simulink model "Pacemaker_A2"  (R2022b)
settings: Solver=FixedStepAuto  StartTime=0.0  StopTime=10.0  FixedStep=1e-3  RelTol=1e-3  EnableMultiTasking=on
undefined symbols (not defined in the file): A0, A1, D0, D1, D10, D11, D12, D13, D2, D3, D5, D6, D8, D9, magnitude, PTA0, PTA1, PTA2, PTB2, PTB3, PTB9, PTC16, PTC17, PTC2, PTC4, PTD0, PTD1, PTD2, PTD3
libraries: frdmk64flib x19, etargetslib x18, dspstat3 x1
settings Model: SimulationMode=external  ExtModeTrigDuration=5  Creator=27161  LastModifiedBy=27161
settings SolverCC: AlgebraicLoopSolver=TrustRegion
settings OptimizationCC: EnhancedBackFolding=on  PassReuseOutputArgsAs=Individual arguments  ZeroExternalMemoryAtStartup=off  ZeroInternalMemoryAtStartup=off  MaxStackSize=64  OptimizeBlockOrder=speed  DifferentSizesBufferReuse=on  OptimizationCustomize=off  EfficientTunableParamExpr=on
settings DebuggingCC: ParameterTunabilityLossMsg=error  UnconnectedInputMsg=warning  UnconnectedOutputMsg=warning  UnconnectedLineMsg=warning  SFMachineParentedDataDiag=warning
settings HardwareCC: ProdBitPerPointer=32  ProdBitPerSizeT=32  ProdBitPerPtrDiffT=32  ProdLargestAtomicInteger=Long  ProdLargestAtomicFloat=Double  ProdWordSize=32  ProdHWDeviceType=ARM Compatible->ARM Cortex
settings ModelReferenceCC: EnableRefExpFcnMdlSchedulingChecks=on
settings SFSimCC: MATLABDynamicMemAlloc=off
settings RTWCC: Description=Embedded Coder  SystemTargetFile=ert.tlc  HardwareBoard=NXP FRDM-K64F  TLCOptions="-aInlineSetEventsForThisBaseRateFcn=TLC_FALSE -aSuppressMultiTaskScheduler=TLC_FALSE  -aRateBasedStepFcn=0"  TemplateMakefile=ert_default_tmf  Toolchain=GNU Tools for ARM Embedded Processors
settings CodeAppCC: ForceParamTrailComments=on  IgnoreCustomStorageClasses=off  OperatorAnnotations=on  SimulinkDataObjDesc=on  SFDataObjDesc=on  InsertBlockDesc=on
settings ERTTargetCC: ExtMode=on  ExtModeTransport=4  ExtModeMexFile=sendToCommService  ExtModeMexArgs='Pacemaker_A2' 0

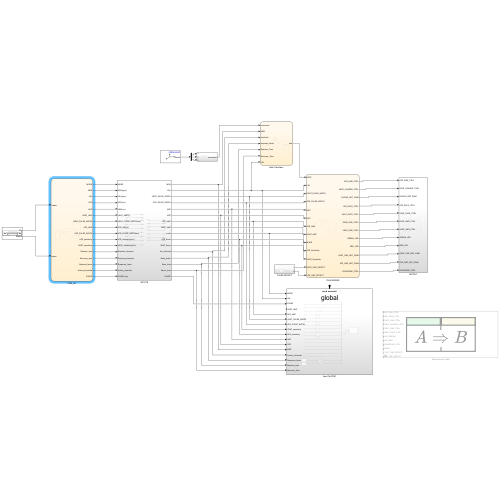
[thumbnail: Simulink's stored preview of the top-level diagram]
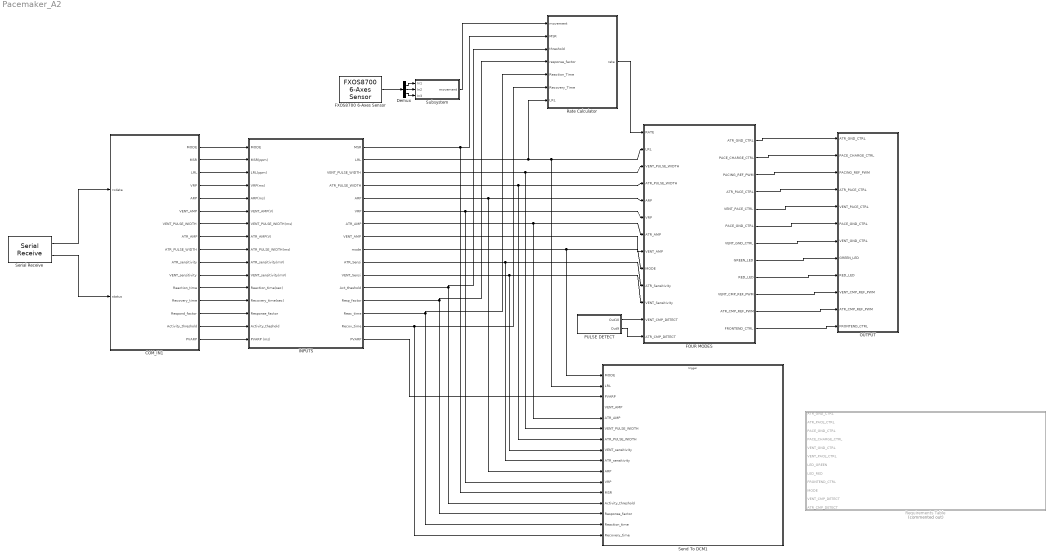
== system Pacemaker_A2 ==
  COM_IN1 : Stateflow chart  TreatAsAtomicUnit=on
      settings: PortSchema="{\"entries\":[{\"content\":{\"sides\":[{\"content\":{\"connectorIds\":[\"In1\",\"In2\"]},\"type\":\"ConnectorPlacement.EquallySpacedRectSide\",\"uuid\":\"bacdf752-87eb-4404-babc-2d3eecd8d2c0\"},{\"content\":{\"connectorIds\":[\"Out12\",\"Out8\",\"Out1\",\"Out2\",\"Out3\",\"Out4\",\"Out5\",\"Out6\",\"Out7\",\"Out9\",\"Out10\",\"Out13\",\"Out14\",\"Out15\",\"Out16\",\"Out11\"],\"side\":\"RIGHT\"},\"type\":\"ConnectorPlacement.EquallySpacedRectSide\",\"uuid\":\"87a5995d-41f9-45bd-b026-59ec7d01c35a\"},{\"content\":{\"connectorIds\":[],\"side\":\"TOP\"},\"type\":\"ConnectorPlacement.EquallySpacedRectSide\",\"uuid\":\"9c1d1ff9-71c1-4ac7-ac77-ae13538ca481\"}]},\"type\":\"ConnectorPlacement.EquallySpacedConnector\",\"uuid\":\"f58684e7-fbf2-4992-a059-d31a56d65e02\"}],\"packageUris\":[\"http://schema.mathworks.com/mf0/Connector/R2020b\"],\"version\":\"1.0\"}"
  Demux : Demux  Outputs=3
  FOUR MODES : Stateflow chart  TreatAsAtomicUnit=on
      settings: PortSchema="{\"entries\":[{\"content\":{\"sides\":[{\"content\":{\"connectorIds\":[\"In11\",\"In8\",\"In2\",\"In1\",\"In9\",\"In10\",\"In5\",\"In4\",\"In6\",\"In13\",\"In12\",\"In3\",\"In7\"]},\"type\":\"ConnectorPlacement.EquallySpacedRectSide\",\"uuid\":\"6661be6b-aedb-4592-878a-fd9116f5820d\"},{\"content\":{\"connectorIds\":[\"Out7\",\"Out1\",\"Out2\",\"Out3\",\"Out4\",\"Out6\",\"Out5\",\"Out9\",\"Out10\",\"Out11\",\"Out12\",\"Out8\"],\"side\":\"RIGHT\"},\"type\":\"ConnectorPlacement.EquallySpacedRectSide\",\"uuid\":\"f16586c3-0c99-4971-ba5f-75b93d25059c\"},{\"content\":{\"connectorIds\":[],\"side\":\"TOP\"},\"type\":\"ConnectorPlacement.EquallySpacedRectSide\",\"uuid\":\"27cb1bd0-c170-4ecc-a4df-3797e7aecef3\"}]},\"type\":\"ConnectorPlacement.EquallySpacedConnector\",\"uuid\":\"03557791-41f4-4916-8cde-1fcab0cf663d\"}],\"packageUris\":[\"http://schema.mathworks.com/mf0/Connector/R2020b\"],\"version\":\"1.0\"}"
  FXOS8700 6-Axes Sensor : frdmk64flib/FXOS8700 6-Axes Sensor  Activesensor=Accelerometer only  ODR=800Hz  HybridODR=400Hz  Accelfullrange=-4g to +4g  SampleTime=-1
  INPUTS : Subsystem
  OUTPUT : Subsystem
  PULSE DETECT : Subsystem
  Rate Calculator : Stateflow chart  TreatAsAtomicUnit=on
      settings: PortSchema="{\"entries\":[{\"content\":{\"sides\":[{\"content\":{\"connectorIds\":[\"In3\",\"In7\",\"In5\",\"In4\",\"In1\",\"In2\",\"In6\"]},\"type\":\"ConnectorPlacement.EquallySpacedRectSide\",\"uuid\":\"c5d5357b-99af-427e-a4c2-6249b97164da\"},{\"content\":{\"connectorIds\":[\"Out1\"],\"side\":\"RIGHT\"},\"type\":\"ConnectorPlacement.EquallySpacedRectSide\",\"uuid\":\"358f3739-9c7f-4556-a3f3-e36ee066d1ea\"},{\"content\":{\"connectorIds\":[],\"side\":\"TOP\"},\"type\":\"ConnectorPlacement.EquallySpacedRectSide\",\"uuid\":\"e7873f65-b91d-40fa-bd89-8dce436ca138\"}]},\"type\":\"ConnectorPlacement.EquallySpacedConnector\",\"uuid\":\"f1b9a7e0-0d96-4ba5-9c87-c58b64bb2144\"}],\"packageUris\":[\"http://schema.mathworks.com/mf0/Connector/R2020b\"],\"version\":\"1.0\"}"
  Requirements Table : Requirements Table  Commented=on  TreatAsAtomicUnit=on
  Send To DCM1 : Subsystem
  Serial Receive : frdmk64flib/Serial Receive  SCIModule=0  Baudrate=uint32(9600)  Parity=None  StopBits=1  HardwareFlowControl=None  ByteOrder=LittleEndian  DataType=uint8  DataLength=10  BlockingMode=off  OutputStatus=on  SampleTime=0.1
  Subsystem : Subsystem
  wires:
  FOUR MODES/7(ATR_GND_CTRL) -> OUTPUT/1(ATR_GND_CTRL)
  FOUR MODES/1(PACE_CHARGE_CTRL) -> OUTPUT/2(PACE_CHARGE_CTRL)
  FOUR MODES/2(PACING_REF_PWM) -> OUTPUT/3(PACING_REF_PWM)
  FOUR MODES/3(ATR_PACE_CTRL) -> OUTPUT/4(ATR_PACE_CTRL)
  FOUR MODES/4(VENT_PACE_CTRL) -> OUTPUT/5(VENT_PACE_CTRL)
  FOUR MODES/5(VENT_GND_CTRL) -> OUTPUT/7(VENT_GND_CTRL)
  FOUR MODES/6(PACE_GND_CTRL) -> OUTPUT/6(PACE_GND_CTRL)
  FOUR MODES/9(GREEN_LED) -> OUTPUT/8(GREEN_LED)
  FOUR MODES/12(ATR_CMP_REF_PWM) -> OUTPUT/11(ATR_CMP_REF_PWM)
  FOUR MODES/11(VENT_CMP_REF_PWM) -> OUTPUT/10(VENT_CMP_REF_PWM)
  FOUR MODES/10(RED_LED) -> OUTPUT/9(RED_LED)
  FOUR MODES/8(FRONTEND_CTRL) -> OUTPUT/12(FRONTEND_CTRL)
  PULSE DETECT/2(Out9) -> FOUR MODES/7(ATR_CMP_DETECT)
  PULSE DETECT/1(Out10) -> FOUR MODES/3(VENT_CMP_DETECT)
  Demux/3 -> Subsystem/3(In3)
  Subsystem/1(movement) -> Rate Calculator/3(movement)
  Demux/1 -> Subsystem/1(In1)
  FXOS8700 6-Axes Sensor/1 -> Demux/1
  Demux/2 -> Subsystem/2(In2)
  COM_IN1/12(MODE) -> INPUTS/1(MODE)
  COM_IN1/1(LRL) -> INPUTS/3(LRL(ppm))
  COM_IN1/2(VRP) -> INPUTS/4(VRP(ms))
  COM_IN1/3(ARP) -> INPUTS/5(ARP(ms))
  COM_IN1/4(VENT_AMP) -> INPUTS/6(VENT_AMP(V))
  COM_IN1/5(VENT_PULSE_WIDTH) -> INPUTS/7(VENT_PULSE_WIDTH(ms))
  COM_IN1/6(ATR_AMP) -> INPUTS/8(ATR_AMP(V))
  COM_IN1/7(ATR_PULSE_WIDTH) -> INPUTS/9(ATR_PULSE_WIDTH(ms))
  COM_IN1/8(MSR) -> INPUTS/2(MSR(ppm))
  COM_IN1/9(ATR_sensitivity) -> INPUTS/10(ATR_sensitivity(mV))
  COM_IN1/10(VENT_sensitivity) -> INPUTS/11(VENT_sensitivity(mV))
  COM_IN1/13(Reaction_time) -> INPUTS/12(Reaction_time(sec))
  COM_IN1/14(Recovery_time) -> INPUTS/13(Recovery_time(sec))
  COM_IN1/11(PVARP) -> INPUTS/16(PVARP (ms))
  Serial Receive/1 -> COM_IN1/1(rxdata)
  Serial Receive/2 -> COM_IN1/2(status)
  COM_IN1/15(Respond_factor) -> INPUTS/14(Response_factor)
  COM_IN1/16(Activity_threshold) -> INPUTS/15(Activity_theshold)
  INPUTS/2(LRL) -> FOUR MODES/8(LRL), Send To DCM1/2(LRL), Rate Calculator/6(LRL)
  INPUTS/1(MSR) -> Rate Calculator/7(MSR), Send To DCM1/12(MSR)
  INPUTS/3(VENT_PULSE_WIDTH) -> FOUR MODES/2(VENT_PULSE_WIDTH), Send To DCM1/6(VENT_PULSE_WIDTH)
  INPUTS/4(ATR_PULSE_WIDTH) -> FOUR MODES/1(ATR_PULSE_WIDTH), Send To DCM1/7(ATR_PULSE_WIDTH)
  INPUTS/5(ARP) -> Send To DCM1/10(ARP), FOUR MODES/9(ARP)
  INPUTS/6(VRP) -> Send To DCM1/11(VRP), FOUR MODES/10(VRP)
  INPUTS/7(ATR_AMP) -> Send To DCM1/5(ATR_AMP), FOUR MODES/5(ATR_AMP)
  INPUTS/8(VENT_AMP) -> FOUR MODES/4(VENT_AMP)
  INPUTS/9(mode) -> Send To DCM1/1(MODE), FOUR MODES/6(MODE)
  INPUTS/14(Reac_time) -> Rate Calculator/1(Reaction_Time), Send To DCM1/15(Reaction_time)
  INPUTS/15(Recov_time) -> Rate Calculator/2(Recovery_Time), Send To DCM1/16(Recovery_time)
  INPUTS/12(Act_theshold) -> Rate Calculator/5(threshold), Send To DCM1/13(Activity_threshold)
  INPUTS/13(Resp_factor) -> Rate Calculator/4(response_factor), Send To DCM1/14(Response_factor)
  INPUTS/10(ATR_Sensi) -> Send To DCM1/9(ATR_sensitivity), FOUR MODES/13(ATR_Sensitivity)
  INPUTS/11(VENT_Sensi) -> Send To DCM1/8(VENT_sensitivity), FOUR MODES/12(VENT_Sensitivity)
  Rate Calculator/1(rate) -> FOUR MODES/11(RATE)
  INPUTS/16(PVARP) -> Send To DCM1/3(PVARP)

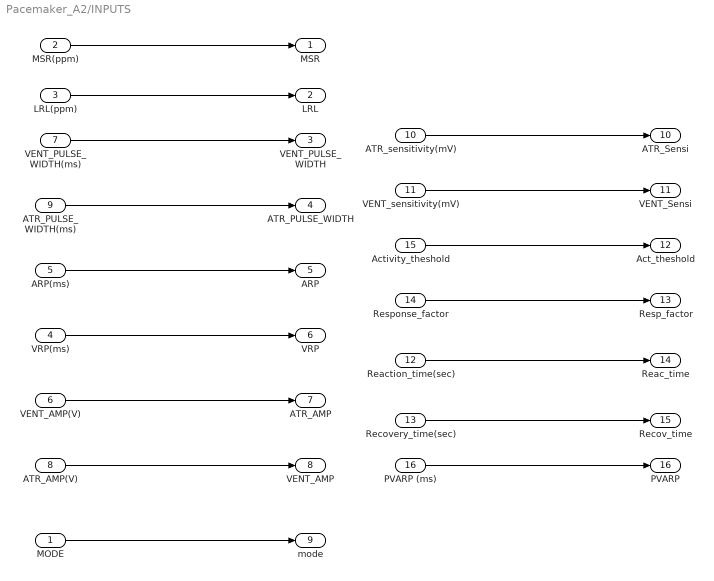
== system Pacemaker_A2/INPUTS ==
  MODE : Inport
  MSR(ppm) : Inport  Port=2
  LRL(ppm) : Inport  Port=3
  VRP(ms) : Inport  Port=4
  ARP(ms) : Inport  Port=5
  VENT_AMP(V) : Inport  Port=6
  VENT_PULSE_WIDTH(ms) : Inport  Port=7
  ATR_AMP(V) : Inport  Port=8
  ATR_PULSE_WIDTH(ms) : Inport  Port=9
  ATR_sensitivity(mV) : Inport  Port=10
  VENT_sensitivity(mV) : Inport  Port=11
  Reaction_time(sec) : Inport  Port=12
  Recovery_time(sec) : Inport  Port=13
  Response_factor : Inport  Port=14
  Activity_theshold : Inport  Port=15
  PVARP (ms) : Inport  Port=16
  MSR : Outport
  LRL : Outport  Port=2
  VENT_PULSE_WIDTH : Outport  Port=3
  ATR_PULSE_WIDTH : Outport  Port=4
  ARP : Outport  Port=5
  VRP : Outport  Port=6
  ATR_AMP : Outport  Port=7
  VENT_AMP : Outport  Port=8
  mode : Outport  Port=9
  ATR_Sensi : Outport  Port=10
  VENT_Sensi : Outport  Port=11
  Act_theshold : Outport  Port=12
  Resp_factor : Outport  Port=13
  Reac_time : Outport  Port=14
  Recov_time : Outport  Port=15
  PVARP : Outport  Port=16
  wires:
  LRL(ppm)/1 -> LRL/1
  VENT_PULSE_WIDTH(ms)/1 -> VENT_PULSE_WIDTH/1
  ATR_PULSE_WIDTH(ms)/1 -> ATR_PULSE_WIDTH/1
  ARP(ms)/1 -> ARP/1
  VRP(ms)/1 -> VRP/1
  VENT_AMP(V)/1 -> ATR_AMP/1
  ATR_AMP(V)/1 -> VENT_AMP/1
  MODE/1 -> mode/1
  MSR(ppm)/1 -> MSR/1
  ATR_sensitivity(mV)/1 -> ATR_Sensi/1
  VENT_sensitivity(mV)/1 -> VENT_Sensi/1
  Activity_theshold/1 -> Act_theshold/1
  Response_factor/1 -> Resp_factor/1
  Reaction_time(sec)/1 -> Reac_time/1
  Recovery_time(sec)/1 -> Recov_time/1
  PVARP (ms)/1 -> PVARP/1

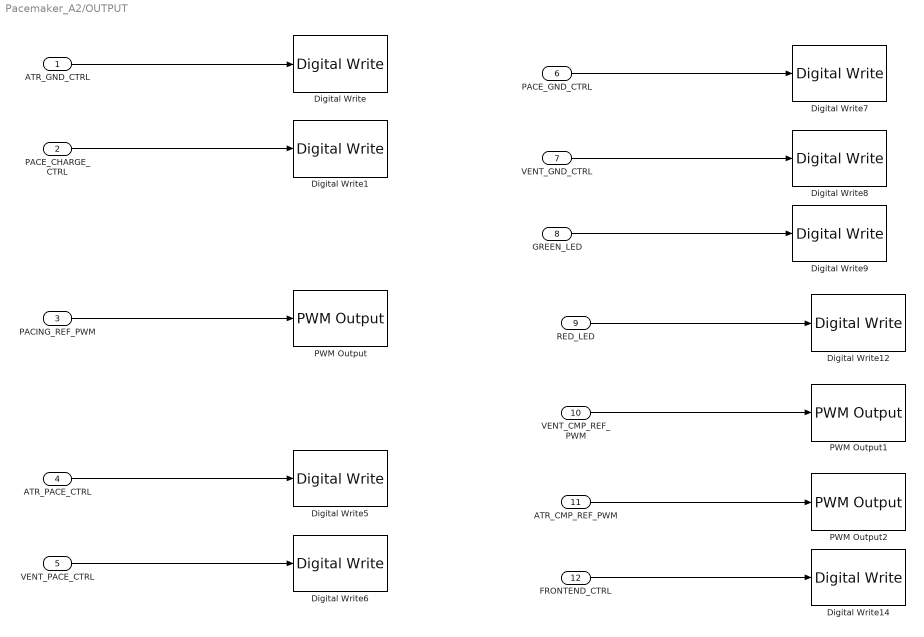
== system Pacemaker_A2/OUTPUT ==
  ATR_GND_CTRL : Inport
  PACE_CHARGE_CTRL : Inport  Port=2
  PACING_REF_PWM : Inport  Port=3
  ATR_PACE_CTRL : Inport  Port=4
  VENT_PACE_CTRL : Inport  Port=5
  PACE_GND_CTRL : Inport  Port=6
  VENT_GND_CTRL : Inport  Port=7
  GREEN_LED : Inport  Port=8
  RED_LED : Inport  Port=9
  VENT_CMP_REF_PWM : Inport  Port=10
  ATR_CMP_REF_PWM : Inport  Port=11
  FRONTEND_CTRL : Inport  Port=12
  Digital Write : frdmk64flib/Digital Write  Whichpin=PTD2 (D11)
  Digital Write1 : frdmk64flib/Digital Write  Whichpin=PTB9 (D2)
  Digital Write12 : frdmk64flib/Digital Write  Whichpin=RED_LED
  Digital Write14 : frdmk64flib/Digital Write  Whichpin=PTD1 (D13)
  Digital Write5 : frdmk64flib/Digital Write  Whichpin=PTA0 (D8)
  Digital Write6 : frdmk64flib/Digital Write  Whichpin=PTC4 (D9)
  Digital Write7 : frdmk64flib/Digital Write  Whichpin=PTD0 (D10)
  Digital Write8 : frdmk64flib/Digital Write  Whichpin=PTD3 (D12)
  Digital Write9 : frdmk64flib/Digital Write  Whichpin=GREEN_LED
  PWM Output : frdmk64flib/PWM Output  Whichpin=PTA2 (D5)  InitialFrequency=2000  InitialDutyCycle=0
  PWM Output1 : frdmk64flib/PWM Output  Whichpin=PTA1 (D3)  InitialFrequency=2000  InitialDutyCycle=0
  PWM Output2 : frdmk64flib/PWM Output  Whichpin=PTC2 (D6)  InitialFrequency=2000  InitialDutyCycle=0
  wires:
  ATR_GND_CTRL/1 -> Digital Write/1
  PACE_CHARGE_CTRL/1 -> Digital Write1/1
  PACING_REF_PWM/1 -> PWM Output/1
  ATR_PACE_CTRL/1 -> Digital Write5/1
  VENT_PACE_CTRL/1 -> Digital Write6/1
  PACE_GND_CTRL/1 -> Digital Write7/1
  VENT_GND_CTRL/1 -> Digital Write8/1
  GREEN_LED/1 -> Digital Write9/1
  ATR_CMP_REF_PWM/1 -> PWM Output2/1
  VENT_CMP_REF_PWM/1 -> PWM Output1/1
  RED_LED/1 -> Digital Write12/1
  FRONTEND_CTRL/1 -> Digital Write14/1

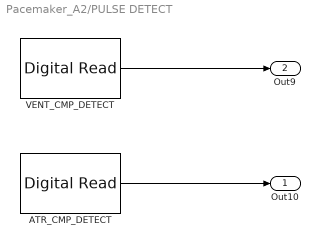
== system Pacemaker_A2/PULSE DETECT ==
  ATR_CMP_DETECT : frdmk64flib/Digital Read  Whichpin=PTC16 (D0)  SampleTime=-1
  VENT_CMP_DETECT : frdmk64flib/Digital Read  Whichpin=PTC17 (D1)  SampleTime=-1
  Out10 : Outport
  Out9 : Outport  Port=2
  wires:
  VENT_CMP_DETECT/1 -> Out9/1
  ATR_CMP_DETECT/1 -> Out10/1

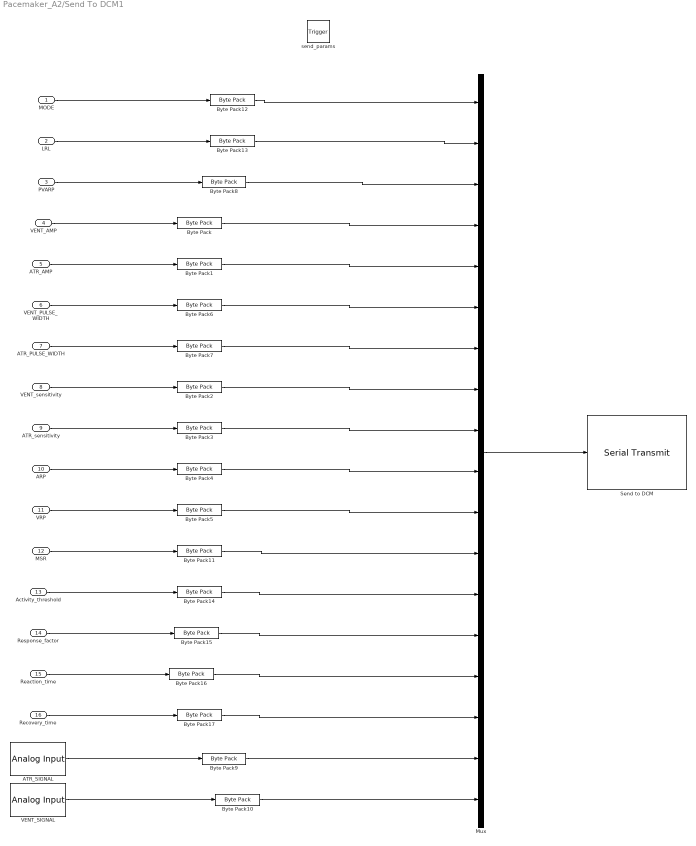
== system Pacemaker_A2/Send To DCM1 ==
  MODE : Inport
  LRL : Inport  Port=2
  PVARP : Inport  Port=3
  VENT_AMP : Inport  Port=4
  ATR_AMP : Inport  Port=5
  VENT_PULSE_WIDTH : Inport  Port=6
  ATR_PULSE_WIDTH : Inport  Port=7
  VENT_sensitivity : Inport  Port=8
  ATR_sensitivity : Inport  Port=9
  ARP : Inport  Port=10
  VRP : Inport  Port=11
  MSR : Inport  Port=12
  Activity_threshold : Inport  Port=13
  Response_factor : Inport  Port=14
  Reaction_time : Inport  Port=15
  Recovery_time : Inport  Port=16
  send_params : TriggerPort  TriggerType=function-call  IsSimulinkFunction=on  FunctionName=send_params  VariantControl=(inherit)  PortDimensions=1
  ATR_SIGNAL : frdmk64flib/Analog Input  Whichpin=PTB2 (A0)  SampleTime=-1
  Byte Pack{,1..3,6..7} (6 alike) : etargetslib/Byte Pack  datatypes={'single'}  byteAlign=1
  Byte Pack10 : etargetslib/Byte Pack  datatypes={'double'}  byteAlign=1
  Byte Pack{4..5,8,11..17} (10 alike) : etargetslib/Byte Pack  datatypes={'uint16'}  byteAlign=1
  Byte Pack9 : etargetslib/Byte Pack  datatypes={'double'}  byteAlign=1
  Mux : Mux  Inputs=18
  Send to DCM : frdmk64flib/Serial Transmit  SCIModule=0  Baudrate=uint32(9600)  Parity=None  StopBits=1  HardwareFlowControl=None  ByteOrder=LittleEndian  BlockingMode=on  OutputStatus=off
  VENT_SIGNAL : frdmk64flib/Analog Input  Whichpin=PTB3 (A1)  SampleTime=-1
  wires:
  MODE/1 -> Byte Pack12/1
  LRL/1 -> Byte Pack13/1
  VENT_AMP/1 -> Byte Pack/1
  Byte Pack/1 -> Mux/4
  ATR_AMP/1 -> Byte Pack1/1
  Byte Pack1/1 -> Mux/5
  VENT_PULSE_WIDTH/1 -> Byte Pack6/1
  ATR_PULSE_WIDTH/1 -> Byte Pack7/1
  VENT_sensitivity/1 -> Byte Pack2/1
  Byte Pack2/1 -> Mux/8
  ATR_sensitivity/1 -> Byte Pack3/1
  Byte Pack3/1 -> Mux/9
  Byte Pack4/1 -> Mux/10
  ARP/1 -> Byte Pack4/1
  VRP/1 -> Byte Pack5/1
  Byte Pack5/1 -> Mux/11
  MSR/1 -> Byte Pack11/1
  Activity_threshold/1 -> Byte Pack14/1
  Response_factor/1 -> Byte Pack15/1
  Reaction_time/1 -> Byte Pack16/1
  Recovery_time/1 -> Byte Pack17/1
  Mux/1 -> Send to DCM/1
  Byte Pack6/1 -> Mux/6
  Byte Pack7/1 -> Mux/7
  PVARP/1 -> Byte Pack8/1
  ATR_SIGNAL/1 -> Byte Pack9/1
  VENT_SIGNAL/1 -> Byte Pack10/1
  Byte Pack10/1 -> Mux/18
  Byte Pack8/1 -> Mux/3
  Byte Pack9/1 -> Mux/17
  Byte Pack12/1 -> Mux/1
  Byte Pack13/1 -> Mux/2
  Byte Pack11/1 -> Mux/12
  Byte Pack14/1 -> Mux/13
  Byte Pack15/1 -> Mux/14
  Byte Pack16/1 -> Mux/15
  Byte Pack17/1 -> Mux/16

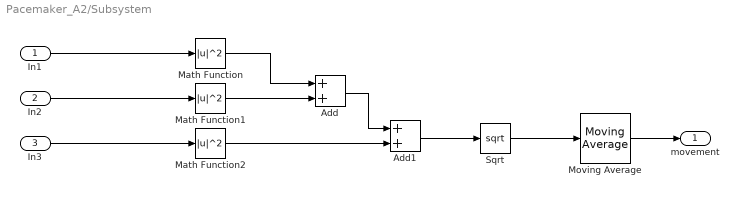
== system Pacemaker_A2/Subsystem ==
  In1 : Inport
  In2 : Inport  Port=2
  In3 : Inport  Port=3
  Add : Sum
  Add1 : Sum
  Math Function : Math  Operator=magnitude^2
  Math Function1 : Math  Operator=magnitude^2
  Math Function2 : Math  Operator=magnitude^2
  Moving Average : dspstat3/Moving Average  Method=Sliding window  ForgettingFactorPort=off  SpecifyWindowLength=on  WindowLength=500  OverlapLength=3  AllowArbitraryInputLength=off  ForgettingFactor=0.9  SimulateUsing=Code generation
  Sqrt : Sqrt
  movement : Outport
  wires:
  In1/1 -> Math Function/1
  Math Function/1 -> Add/1
  In2/1 -> Math Function1/1
  Math Function1/1 -> Add/2
  In3/1 -> Math Function2/1
  Math Function2/1 -> Add1/2
  Add/1 -> Add1/1
  Add1/1 -> Sqrt/1
  Sqrt/1 -> Moving Average/1
  Moving Average/1 -> movement/1

== stateflow chart Pacemaker_A2/Requirements Table ==
  (default) -> (junction 1073751917)
  (junction 1073751917) -> (junction 1073751918) : {
      | % SF_REQ_REV_07
      | }
  (junction 1073751918) -> (junction 1073751920) : {
      | % HEADER_ASSIGNMENTS
      |
      | }
  (junction 1073751920) -> (junction 1073751922) : {
      | % START_A_4
      | }
  (junction 1073751922) -> (junction 1073751924) : {
      | }
  (junction 1073751924) -> (junction 1073751926)
  (junction 1073751926) -> (junction 1073751928) : {
      | }
  (junction 1073751928) -> (junction 1073751930) : {
      | % END_A_4
      | }
  (junction 1073751930) -> (junction 1073751932) : {
      | % START_R_1
      | }
  (junction 1073751932) -> (junction 1073751934) : {
      | }
  (junction 1073751934) -> (junction 1073751936)
  (junction 1073751936) -> (junction 1073751938) [order 1] : [(((MODE) == (1)))]
  (junction 1073751936) -> (junction 1073751980) [order 2]
  (junction 1073751938) -> (junction 1073751940) : {
      |
      |
      | }
  (junction 1073751940) -> (junction 1073751942) : {
      | }
  (junction 1073751942) -> (junction 1073751944) : {
      | % START_R_7
      | }
  (junction 1073751944) -> (junction 1073751946) : {
      | }
  (junction 1073751946) -> (junction 1073751948)
  (junction 1073751948) -> (junction 1073751950) [order 1] : [(((state) == (1)))]
  (junction 1073751948) -> (junction 1073751956) [order 2]
  (junction 1073751950) -> (junction 1073751952) : {
      | reqtable_postcondition((((PACE_GND_CTRL) == (true))) && (((PACE_CHARGE_CTRL) == (false))) && (((ATR_GND_CTRL) == (false))) && (((ATR_PACE_CTRL) == (true))) && (((LED_GREEN) == (false))), 'R:1.1');
      |
      |
      | }
  (junction 1073751952) -> (junction 1073751954) : {
      | }
  (junction 1073751954) -> (junction 1073751956)
  (junction 1073751956) -> (junction 1073751958)
  (junction 1073751958) -> (junction 1073751960) : {
      | % END_R_7
      | }
  (junction 1073751960) -> (junction 1073751962) : {
      | % START_R_34
      | }
  (junction 1073751962) -> (junction 1073751964) : {
      | }
  (junction 1073751964) -> (junction 1073751966)
  (junction 1073751966) -> (junction 1073751968) [order 1] : [(((state) == (2)))]
  (junction 1073751966) -> (junction 1073751974) [order 2]
  (junction 1073751968) -> (junction 1073751970) : {
      | reqtable_postcondition((((PACE_GND_CTRL) == (true))) && (((PACE_CHARGE_CTRL) == (true))) && (((ATR_GND_CTRL) == (true))) && (((ATR_PACE_CTRL) == (false))) && (((LED_GREEN) == (true))), 'R:1.2');
      |
      |
      | }
  (junction 1073751970) -> (junction 1073751972) : {
      | }
  (junction 1073751972) -> (junction 1073751974)
  (junction 1073751974) -> (junction 1073751976)
  (junction 1073751976) -> (junction 1073751978) : {
      | % END_R_34
      | }
  (junction 1073751978) -> (junction 1073751980)
  (junction 1073751980) -> (junction 1073751982)
  (junction 1073751982) -> (junction 1073751984) : {
      | % END_R_1
      | }
  (junction 1073751984) -> (junction 1073751986) : {
      | % START_R_10
      | }
  (junction 1073751986) -> (junction 1073751988) : {
      | }
  (junction 1073751988) -> (junction 1073751990)
  (junction 1073751990) -> (junction 1073751992) [order 1] : [(((MODE) == (2)))]
  (junction 1073751990) -> (junction 1073752034) [order 2]
  (junction 1073751992) -> (junction 1073751994) : {
      |
      |
      | }
  (junction 1073751994) -> (junction 1073751996) : {
      | }
  (junction 1073751996) -> (junction 1073751998) : {
      | % START_R_28
      | }
  (junction 1073751998) -> (junction 1073752000) : {
      | }
  (junction 1073752000) -> (junction 1073752002)
  (junction 1073752002) -> (junction 1073752004) [order 1] : [(((state) == (1)))]
  (junction 1073752002) -> (junction 1073752010) [order 2]
  (junction 1073752004) -> (junction 1073752006) : {
      | reqtable_postcondition((((PACE_GND_CTRL) == (true))) && (((PACE_CHARGE_CTRL) == (false))) && (((VENT_PACE_CTRL) == (true))) && (((VENT_GND_CTRL) == (false))) && (((LED_RED) == (false))), 'R:2.1');
      |
      |
      | }
  (junction 1073752006) -> (junction 1073752008) : {
      | }
  (junction 1073752008) -> (junction 1073752010)
  (junction 1073752010) -> (junction 1073752012)
  (junction 1073752012) -> (junction 1073752014) : {
      | % END_R_28
      | }
  (junction 1073752014) -> (junction 1073752016) : {
      | % START_R_31
      | }
  (junction 1073752016) -> (junction 1073752018) : {
      | }
  (junction 1073752018) -> (junction 1073752020)
  (junction 1073752020) -> (junction 1073752022) [order 1] : [(((state) == (2)))]
  (junction 1073752020) -> (junction 1073752028) [order 2]
  (junction 1073752022) -> (junction 1073752024) : {
      | reqtable_postcondition((((PACE_GND_CTRL) == (true))) && (((PACE_CHARGE_CTRL) == (true))) && (((VENT_PACE_CTRL) == (false))) && (((VENT_GND_CTRL) == (true))) && (((LED_RED) == (true))), 'R:2.2');
      |
      |
      | }
  (junction 1073752024) -> (junction 1073752026) : {
      | }
  (junction 1073752026) -> (junction 1073752028)
  (junction 1073752028) -> (junction 1073752030)
  (junction 1073752030) -> (junction 1073752032) : {
      | % END_R_31
      | }
  (junction 1073752032) -> (junction 1073752034)
  (junction 1073752034) -> (junction 1073752036)
  (junction 1073752036) -> (junction 1073752038) : {
      | % END_R_10
      | }
  (junction 1073752038) -> (junction 1073752040) : {
      | % START_R_13
      | }
  (junction 1073752040) -> (junction 1073752042) : {
      | }
  (junction 1073752042) -> (junction 1073752044)
  (junction 1073752044) -> (junction 1073752046) [order 1] : [(((MODE) == (3)))]
  (junction 1073752044) -> (junction 1073752106) [order 2]
  (junction 1073752046) -> (junction 1073752048) : {
      |
      |
      | }
  (junction 1073752048) -> (junction 1073752050) : {
      | }
  (junction 1073752050) -> (junction 1073752052) : {
      | % START_R_19
      | }
  (junction 1073752052) -> (junction 1073752054) : {
      | }
  (junction 1073752054) -> (junction 1073752056)
  (junction 1073752056) -> (junction 1073752058) [order 1] : [(((state) == (1)))]
  (junction 1073752056) -> (junction 1073752064) [order 2]
  (junction 1073752058) -> (junction 1073752060) : {
      | reqtable_postcondition((((PACE_GND_CTRL) == (true))) && (((PACE_CHARGE_CTRL) == (true))) && (((VENT_PACE_CTRL) == (false))) && (((VENT_GND_CTRL) == (true))) && (((FRONTEND_CTRL) == (true))) && (((LED_RED) == (true))), 'R:3.1');
      |
      |
      | }
  (junction 1073752060) -> (junction 1073752062) : {
      | }
  (junction 1073752062) -> (junction 1073752064)
  (junction 1073752064) -> (junction 1073752066)
  (junction 1073752066) -> (junction 1073752068) : {
      | % END_R_19
      | }
  (junction 1073752068) -> (junction 1073752070) : {
      | % START_R_22
      | }
  (junction 1073752070) -> (junction 1073752072) : {
      | }
  (junction 1073752072) -> (junction 1073752074)
  (junction 1073752074) -> (junction 1073752076) [order 1] : [(((state) == (2)))]
  (junction 1073752074) -> (junction 1073752082) [order 2]
  (junction 1073752076) -> (junction 1073752078) : {
      | reqtable_postcondition((((PACE_GND_CTRL) == (true))) && (((PACE_CHARGE_CTRL) == (false))) && (((VENT_PACE_CTRL) == (true))) && (((VENT_GND_CTRL) == (false))) && (((LED_GREEN) == (true))), 'R:3.2');
      |
      |
      | }
  (junction 1073752078) -> (junction 1073752080) : {
      | }
  (junction 1073752080) -> (junction 1073752082)
  (junction 1073752082) -> (junction 1073752084)
  (junction 1073752084) -> (junction 1073752086) : {
      | % END_R_22
      | }
  (junction 1073752086) -> (junction 1073752088) : {
      | % START_R_43
      | }
  (junction 1073752088) -> (junction 1073752090) : {
      | }
  (junction 1073752090) -> (junction 1073752092)
  (junction 1073752092) -> (junction 1073752094) [order 1] : [(((state) == (3)))]
  (junction 1073752092) -> (junction 1073752100) [order 2]
  (junction 1073752094) -> (junction 1073752096) : {
      | reqtable_postcondition((((PACE_GND_CTRL) == (true))) && (((PACE_CHARGE_CTRL) == (false))) && (((VENT_PACE_CTRL) == (false))) && (((VENT_GND_CTRL) == (true))) && (((FRONTEND_CTRL) == (false))) && (((LED_RED) == (false))), 'R:3.3');
      |
      |
      | }
  (junction 1073752096) -> (junction 1073752098) : {
      | }
  (junction 1073752098) -> (junction 1073752100)
  (junction 1073752100) -> (junction 1073752102)
  (junction 1073752102) -> (junction 1073752104) : {
      | % END_R_43
      | }
  (junction 1073752104) -> (junction 1073752106)
  (junction 1073752106) -> (junction 1073752108)
  (junction 1073752108) -> (junction 1073752110) : {
      | % END_R_13
      | }
  (junction 1073752110) -> (junction 1073752112) : {
      | % START_R_16
      | }
  (junction 1073752112) -> (junction 1073752114) : {
      | }
  (junction 1073752114) -> (junction 1073752116)
  (junction 1073752116) -> (junction 1073752118) [order 1] : [(((MODE) == (4)))]
  (junction 1073752116) -> (junction 1073752178) [order 2]
  (junction 1073752118) -> (junction 1073752120) : {
      |
      |
      | }
  (junction 1073752120) -> (junction 1073752122) : {
      | }
  (junction 1073752122) -> (junction 1073752124) : {
      | % START_R_37
      | }
  (junction 1073752124) -> (junction 1073752126) : {
      | }
  (junction 1073752126) -> (junction 1073752128)
  (junction 1073752128) -> (junction 1073752130) [order 1] : [(((state) == (1)))]
  (junction 1073752128) -> (junction 1073752136) [order 2]
  (junction 1073752130) -> (junction 1073752132) : {
      | reqtable_postcondition((((PACE_GND_CTRL) == (true))) && (((PACE_CHARGE_CTRL) == (true))) && (((ATR_GND_CTRL) == (true))) && (((ATR_PACE_CTRL) == (false))) && (((FRONTEND_CTRL) == (true))) && (((LED_GREEN) == (true))), 'R:4.1');
      |
      |
      | }
  (junction 1073752132) -> (junction 1073752134) : {
      | }
  (junction 1073752134) -> (junction 1073752136)
  (junction 1073752136) -> (junction 1073752138)
  (junction 1073752138) -> (junction 1073752140) : {
      | % END_R_37
      | }
  (junction 1073752140) -> (junction 1073752142) : {
      | % START_R_40
      | }
  (junction 1073752142) -> (junction 1073752144) : {
      | }
  (junction 1073752144) -> (junction 1073752146)
  (junction 1073752146) -> (junction 1073752148) [order 1] : [(((state) == (2)))]
  (junction 1073752146) -> (junction 1073752154) [order 2]
  (junction 1073752148) -> (junction 1073752150) : {
      | reqtable_postcondition((((PACE_GND_CTRL) == (true))) && (((PACE_CHARGE_CTRL) == (false))) && (((ATR_GND_CTRL) == (false))) && (((ATR_PACE_CTRL) == (true))) && (((LED_RED) == (true))), 'R:4.2');
      |
      |
      | }
  (junction 1073752150) -> (junction 1073752152) : {
      | }
  (junction 1073752152) -> (junction 1073752154)
  (junction 1073752154) -> (junction 1073752156)
  (junction 1073752156) -> (junction 1073752158) : {
      | % END_R_40
      | }
  (junction 1073752158) -> (junction 1073752160) : {
      | % START_R_46
      | }
  (junction 1073752160) -> (junction 1073752162) : {
      | }
  (junction 1073752162) -> (junction 1073752164)
  (junction 1073752164) -> (junction 1073752166) [order 1] : [(((state) == (3)))]
  (junction 1073752164) -> (junction 1073752172) [order 2]
  (junction 1073752166) -> (junction 1073752168) : {
      | reqtable_postcondition((((PACE_GND_CTRL) == (true))) && (((PACE_CHARGE_CTRL) == (false))) && (((ATR_GND_CTRL) == (true))) && (((ATR_PACE_CTRL) == (false))) && (((FRONTEND_CTRL) == (false))) && (((LED_GREEN) == (false))), 'R:4.3');
      |
      |
      | }
  (junction 1073752168) -> (junction 1073752170) : {
      | }
  (junction 1073752170) -> (junction 1073752172)
  (junction 1073752172) -> (junction 1073752174)
  (junction 1073752174) -> (junction 1073752176) : {
      | % END_R_46
      | }
  (junction 1073752176) -> (junction 1073752178)
  (junction 1073752178) -> (junction 1073752180)
  (junction 1073752180) -> (junction 1073752182) : {
      | % END_R_16
      | }
  data: ATR_GND_CTRL input; ATR_PACE_CTRL input; PACE_GND_CTRL input; PACE_CHARGE_CTRL input; VENT_GND_CTRL input; VENT_PACE_CTRL input; LED_GREEN input; LED_RED input; FRONTEND_CTRL input; MODE input; VENT_CMP_DETECT input; ATR_CMP_DETECT input

== stateflow chart Pacemaker_A2/COM_IN1 ==
  note: Waiting for DCM team data order to fill in the rxdata.
  state SET_PARAM
    entry:
    MODE = typecast(rxdata(3:4),'uint16');
    LRL = typecast(rxdata(5:6),'uint16');
    ATR_AMP = typecast(rxdata(7:10), 'single');
    ATR_PULSE_WIDTH = typecast(rxdata(11:14), 'single');
    VENT_AMP = typecast(rxdata(15:18), 'single');
    VENT_PULSE_WIDTH = typecast(rxdata(19:22), 'single');
    VRP = typecast(rxdata(23:24), 'uint16');
    ARP = typecast(rxdata(25:26), 'uint16');
    MSR = typecast(rxdata(27:28), 'uint16');
    ATR_sensitivity =typecast(rxdata(29:32), 'single');
    VENT_sensitivity = typecast(rxdata(33:36) ,'single');
    PVARP = typecast(rxdata(37:38), 'uint16');
    Activity_threshold = typecast(rxdata(39:40), 'uint16');
    Reaction_time = typecast(rxdata(41:42), 'uint16');
    Respond_factor =typecast(rxdata(43:44), 'uint16');
    Recovery_time = typecast(rxdata(45:46), 'uint16');
  state INITIAL
    entry:
    MODE = 1; %select any mode
    LRL = 30; %ppm
    ATR_AMP = 0;
    ATR_PULSE_WIDTH = 0.05;
    VENT_AMP = 0;
    VENT_PULSE_WIDTH = 0.05;
    VRP = 150;
    ARP = 150;
    MSR = 50;
    ATR_sensitivity = 0.25;
    VENT_sensitivity = 0.25;
    PVARP = 150;
    Activity_threshold = 0;
    Reaction_time = 10;
    Respond_factor = 1;
    Recovery_time = 2;
  state STANDBY
    %waiting for COM
  state ECHO_PARAM
    entry:
    send_params();
  SET_PARAM -> STANDBY
  (default) -> INITIAL
  (junction 14) -> SET_PARAM [order 1] : [rxdata(2) == hex2dec('55')]
  INITIAL -> STANDBY
  STANDBY -> (junction 15) : [status == 0]
  (junction 15) -> (junction 14) : [rxdata(1) == hex2dec('16')]
  (junction 14) -> ECHO_PARAM [order 2] : [rxdata(2) == hex2dec('22')]
  ECHO_PARAM -> STANDBY
  data: rxdata input uint8; status input uint8; LRL output uint16; VRP output uint16; ARP output uint16; VENT_AMP output single; VENT_PULSE_WIDTH output single; ATR_AMP output single; ATR_PULSE_WIDTH output single; MSR output uint16; ATR_sensitivity output single; VENT_sensitivity output single; PVARP output uint16; MODE output uint16; Reaction_time output uint16; Recovery_time output uint16; Respond_factor output uint16; Activity_threshold output uint16

== stateflow chart Pacemaker_A2/FOUR MODES ==
  state AAIR
    note: AAIR is almost the same as AAI. The only difference is that we changed LRL to RATE during the trasition to implement adaptive rate.
    state AAIR_INITIAL
      entry:
      FRONTEND_CTRL= true;
      ATR_PACE_CTRL = false;
      PACING_REF_PWM = ATR_AMP/5*100;
      PACE_CHARGE_CTRL = true;
      PACE_GND_CTRL = true;
      ATR_GND_CTRL = true;
      ATR_CMP_REF_PWM = ATR_Sensitivity/3.3*100;
      GREEN_LED = 1;
    state AAIR_PACING
      entry:
      PACE_CHARGE_CTRL = false;
      PACE_GND_CTRL = true;
      ATR_PACE_CTRL = true;
      ATR_GND_CTRL = false;
      RED_LED = 1;
    state AAIR_REF
      entry:
      FRONTEND_CTRL = false;
      ATR_PACE_CTRL = false;
      ATR_GND_CTRL = true;
      ATR_CMP_REF_PWM = ATR_AMP*20;
      PACE_CHARGE_CTRL = false;
      PACE_GND_CTRL = true;
      GREEN_LED = 0;
    (default) -> AAIR_INITIAL
    AAIR_INITIAL -> AAIR_PACING [order 1] : [(ATR_CMP_DETECT == false) && after(60000/RATE - ATR_PULSE_WIDTH - ARP,msec)]
    AAIR_REF -> AAIR_INITIAL : [after(ARP, msec)]
    AAIR_INITIAL -> AAIR_REF [order 2] : [ATR_CMP_DETECT == true]
    AAIR_PACING -> AAIR_REF : [after(ATR_PULSE_WIDTH,msec)]
  note: In the AOO initial state, we start charging C22 to prepare to pace.
      | Also, we begin to discharge C21 from the last pace.
  note: In the initial state of AAI, we have
      | sensor on to detact if the input voltage is higher
      | than our set threshlod.
      |
      | We also charge C22 for possible pacing
      | state happen when not detection of natural
      | pulse, and discharge C21 to end the pacing state.
      |
      | LED light is off at initial state.
  state AOO_INITIAL
    entry:
    ATR_PACE_CTRL = false;
    ATR_GND_CTRL = true;
    PACE_CHARGE_CTRL = true;
    PACE_GND_CTRL = true;
    PACING_REF_PWM = ATR_AMP*20
    GREEN_LED = 1;
  state AOO_PACING
    PACE_CHARGE_CTRL = false;
    PACE_GND_CTRL = true;
    ATR_PACE_CTRL = true;
    ATR_GND_CTRL = false;
    GREEN_LED =0;
  state AAI_INITIAL
    entry:
    FRONTEND_CTRL= true;
    ATR_PACE_CTRL = false;
    PACING_REF_PWM = ATR_AMP/5*100;
    PACE_CHARGE_CTRL = true;
    PACE_GND_CTRL = true;
    ATR_GND_CTRL = true;
    ATR_CMP_REF_PWM = ATR_Sensitivity/3.3*100;
    GREEN_LED = 1;
  note: In the MainState, we set all of our set points to 0 and detect which mode we go next.
  note: We have a total cycle of 60s/LRL(BPM)
  state MainState
    entry:
    ATR_PACE_CTRL = false;
    ATR_GND_CTRL = false;
    VENT_GND_CTRL = false;
    VENT_PACE_CTRL = false;
    PACE_CHARGE_CTRL = false;
    PACE_GND_CTRL = false;
    FRONTEND_CTRL = false;
  note: In the pacing state, we connect C22 to C21 to pace the Atrium
  state AOOR
    note: AOOR is almost the same as AOO. The only difference is that we changed LRL to RATE during the trasition to implement adaptive rate.
    state AOOR_INITIAL
      entry:
      ATR_PACE_CTRL = false;
      ATR_GND_CTRL = true;
      PACE_CHARGE_CTRL = true;
      PACE_GND_CTRL = true;
      PACING_REF_PWM = ATR_AMP*20
      GREEN_LED = 1;
    state AOOR_PACING
      PACE_CHARGE_CTRL = false;
      PACE_GND_CTRL = true;
      ATR_PACE_CTRL = true;
      ATR_GND_CTRL = false;
      GREEN_LED =0;
    (default) -> AOOR_INITIAL
    AOOR_INITIAL -> AOOR_PACING : [after(60000/RATE - ATR_PULSE_WIDTH),msec]
    AOOR_PACING -> AOOR_INITIAL : after(ATR_PULSE_WIDTH,msec)
  state AAI_PACING
    entry:
    PACE_CHARGE_CTRL = false;
    PACE_GND_CTRL = true;
    ATR_PACE_CTRL = true;
    ATR_GND_CTRL = false;
    RED_LED = 1;
  state VOO_INITIAL
    entry:
    VENT_GND_CTRL = true;
    VENT_PACE_CTRL = false;
    PACE_CHARGE_CTRL = true;
    PACE_GND_CTRL = true;
    PACING_REF_PWM = VENT_AMP*20
    RED_LED = 1;
  note: In the VOO initial state, we start charging C22 to prepare to pace.
      | Also, we begin to discharge C21 from the last pace.
  state VOO_PACING
    PACE_CHARGE_CTRL = false;
    PACE_GND_CTRL = true;
    VENT_GND_CTRL = false;
    VENT_PACE_CTRL = true;
    RED_LED =0;
  state AAI_REF
    entry:
    FRONTEND_CTRL = false;
    ATR_PACE_CTRL = false;
    ATR_GND_CTRL = true;
    ATR_CMP_REF_PWM = ATR_AMP*20;
    PACE_CHARGE_CTRL = false;
    PACE_GND_CTRL = true;
    GREEN_LED = 0;
  state VVIR
    note: VVIR is almost the same as VVI. The only difference is that we changed LRL to RATE during the trasition to implement adaptive rate.
    state VVIR_REF
      entry:
      FRONTEND_CTRL = false;
      VENT_PACE_CTRL = false;
      VENT_GND_CTRL = true;
      PACING_REF_PWM = VENT_AMP*20;
      PACE_CHARGE_CTRL = false;
      PACE_GND_CTRL = true;
      RED_LED = 0;
    state VVIR_INITIAL
      entry:
      PACING_REF_PWM = VENT_AMP*20;
      PACE_GND_CTRL = true;
      VENT_GND_CTRL = true;
      VENT_PACE_CTRL = false;
      PACE_CHARGE_CTRL = true;
      VENT_CMP_REF_PWM = VENT_Sensitivity/3.3*100;
      FRONTEND_CTRL= true;
      RED_LED = 1;
    state VVIR_PACING
      entry:
      PACE_CHARGE_CTRL = false;
      PACE_GND_CTRL = true;
      VENT_GND_CTRL = false;
      VENT_PACE_CTRL = true;
      GREEN_LED = 1;
    (default) -> VVIR_INITIAL
    VVIR_REF -> VVIR_INITIAL : [after(VRP, msec)]
    VVIR_INITIAL -> VVIR_REF [order 2] : [VENT_CMP_DETECT == 1]
    VVIR_PACING -> VVIR_REF : [after(VENT_PULSE_WIDTH,msec)]
    VVIR_INITIAL -> VVIR_PACING [order 1] : [(VENT_CMP_DETECT == 0) && after(60000/RATE - VENT_PULSE_WIDTH - VRP,msec)]
  note: When no detect natural pulse, pace the atrium
      | with connecting C22 to C11. Then wait for 1 cycle.
  note: After a pulse width, stop pacing
  state VOOR
    note: VOOR is almost the same as VOO. The only difference is that we changed LRL to RATE during the trasition to implement adaptive rate.
    state VOOR_INTIAL
      entry:
      VENT_GND_CTRL = true;
      VENT_PACE_CTRL = false;
      PACE_CHARGE_CTRL = true;
      PACE_GND_CTRL = true;
      PACING_REF_PWM = VENT_AMP*20
      RED_LED = 1;
    state VOOR_PACING
      PACE_CHARGE_CTRL = false;
      PACE_GND_CTRL = true;
      VENT_GND_CTRL = false;
      VENT_PACE_CTRL = true;
      RED_LED =0;
    (default) -> VOOR_INTIAL
    VOOR_INTIAL -> VOOR_PACING : [after(60000/RATE - VENT_PULSE_WIDTH,msec)]
    VOOR_PACING -> VOOR_INTIAL : [after(VENT_PULSE_WIDTH,msec)]
  note: In the Refractory state, sensor turn off.
      | A signal of this happen will have red LED turn on.
      | After a refractory period, go back to initial state.
  state VVI_REF
    entry:
    FRONTEND_CTRL = false;
    VENT_PACE_CTRL = false;
    VENT_GND_CTRL = true;
    PACING_REF_PWM = VENT_AMP*20;
    PACE_CHARGE_CTRL = false;
    PACE_GND_CTRL = true;
    RED_LED = 0;
  state VVI_INITIAL
    entry:
    PACING_REF_PWM = VENT_AMP*20;
    PACE_GND_CTRL = true;
    VENT_GND_CTRL = true;
    VENT_PACE_CTRL = false;
    PACE_CHARGE_CTRL = true;
    VENT_CMP_REF_PWM = VENT_Sensitivity/3.3*100;
    FRONTEND_CTRL= true;
    RED_LED = 1;
  note: In the Refractory state, sensor turn off.
      | A signal of this happen will have red LED turn on.
      | After a refractory period, go back to initial state.
  note: In the initial state of VVI, we turn the
      | sensor on to detect if the input voltage is higher
      | than our set threshlod.
      |
      | We also charge C22 for possible pacing
      | state happen when not detection of natural
      | pulse, and discharge C21 to end the pacing state.
      |
      | LED light is off at initial state.
  state VVI_PACING
    entry:
    PACE_CHARGE_CTRL = false;
    PACE_GND_CTRL = true;
    VENT_GND_CTRL = false;
    VENT_PACE_CTRL = true;
    GREEN_LED = 1;
  note: Discharging C22 to C21 to pace the ventricle.
      | Same as VOO pacing.
  MainState -> AAIR [order 8] : [MODE == 8]
  AOO_PACING -> AOO_INITIAL : [after(ATR_PULSE_WIDTH,msec)]
  (default) -> MainState
  AOO_INITIAL -> AOO_PACING : [after(60000/LRL - ATR_PULSE_WIDTH,msec)]
  MainState -> AOO_INITIAL [order 2] : [MODE == 1]
  AAI_INITIAL -> AAI_PACING [order 1] : [(ATR_CMP_DETECT == false) && after(60000/LRL - ATR_PULSE_WIDTH - ARP,msec)]
  MainState -> AAI_INITIAL [order 1] : [MODE == 4]
  MainState -> AOOR [order 5] : [MODE == 5]
  AAI_REF -> AAI_INITIAL : [after(ARP, msec)]
  AAI_INITIAL -> AAI_REF [order 2] : [ATR_CMP_DETECT == true]
  MainState -> VVIR [order 7] : [MODE == 7]
  MainState -> VOO_INITIAL [order 3] : [MODE == 2]
  MainState -> VVI_INITIAL [order 4] : [MODE == 3]
  MainState -> VOOR [order 6] : [MODE == 6]
  VOO_INITIAL -> VOO_PACING : [after(60000/LRL - VENT_PULSE_WIDTH,msec)]
  AAI_PACING -> AAI_REF : [after(ATR_PULSE_WIDTH,msec)]
  VOO_PACING -> VOO_INITIAL : [after(VENT_PULSE_WIDTH,msec)]
  VVI_REF -> VVI_INITIAL : [after(VRP, msec)]
  VVI_INITIAL -> VVI_REF [order 2] : [VENT_CMP_DETECT == 1]
  VVI_PACING -> VVI_REF : [after(VENT_PULSE_WIDTH,msec)]
  VVI_INITIAL -> VVI_PACING [order 1] : [(VENT_CMP_DETECT == 0) && after(60000/LRL - VENT_PULSE_WIDTH - VRP,msec)]
  data: PACE_CHARGE_CTRL output; PACING_REF_PWM output; ATR_PACE_CTRL output; VENT_PACE_CTRL output; VENT_GND_CTRL output; PACE_GND_CTRL output; ATR_GND_CTRL output; ATR_PULSE_WIDTH input; VENT_PULSE_WIDTH input; FRONTEND_CTRL output; GREEN_LED output; VENT_CMP_DETECT input; VENT_AMP input; RED_LED output; ATR_AMP input; MODE input; VENT_CMP_REF_PWM output; ATR_CMP_DETECT input; ATR_CMP_REF_PWM output; LRL input; ARP input; VRP input; RATE input; VENT_Sensitivity input; ATR_Sensitivity input

== stateflow chart Pacemaker_A2/Rate Calculator ==
  state Begin
    entry:
    rate = LRL;
  state Reduce
    entry:
    target_rate = LRL;
  state Data_Check
    entry:
    reduce_step_size = (MSR-LRL)/Recovery_Time;
    increase_step_size = (MSR-LRL)/Reaction_Time;
  state Addition
    entry:
    target_rate = LRL+response_factor* (movement-threshold);
    if(target_rate>=MSR)
    target_rate = MSR;
    end
  state Change1
    entry:
    if(rate< target_rate)
    rate = rate+ increase_step_size;
    elseif(rate == target_rate)
    rate = target_rate;
    elseif(rate > target_rate)
    rate = rate - reduce_step_size;
    end
  state Change2
    entry:
    if(rate< target_rate)
    rate = rate+ increase_step_size;
    elseif(rate == target_rate)
    rate = target_rate;
    elseif(rate > target_rate)
    rate = rate - reduce_step_size;
    end
  (default) -> Begin
  Begin -> Data_Check
  Data_Check -> Reduce [order 2] : [movement<threshold]
  Data_Check -> Addition [order 1] : [movement>=threshold]
  Addition -> Data_Check [order 1] : [movement<threshold]
  Reduce -> Data_Check [order 1] : [movement>=threshold]
  Change1 -> Reduce : [after(100,msec)]
  Reduce -> Change1 [order 2] : [after(100,msec)]
  Change2 -> Addition : [after(100,msec)]
  Addition -> Change2 [order 2] : [after(100,msec)]
  data: Reaction_Time input; Recovery_Time input; movement input; rate output; response_factor input; threshold input; LRL input; MSR input; increase_step_size local; target_rate local; reduce_step_size local
